simulink model "LL_rdf0"  (R2013b)
settings: Solver=ode45  StartTime=0.0  StopTime=10.0  RelTol=1e-3
settings Model: Creator=rmg37  LastModifiedBy=rmg37

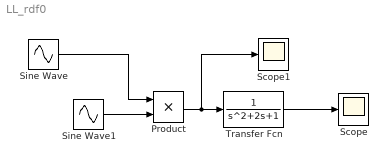
== system LL_rdf0 ==
  Product : Product
  Scope : Scope
  Scope1 : Scope
  Sine Wave : Sin  Frequency=2*pi*99.9  SampleTime=0
  Sine Wave1 : Sin  Frequency=2*pi*100  SampleTime=0
  Transfer Fcn : TransferFcn
  wires:
  Sine Wave/1 -> Product/1
  Sine Wave1/1 -> Product/2
  Product/1 -> Scope1/1, Transfer Fcn/1
  Transfer Fcn/1 -> Scope/1
